simulink model "ROSCO"  (R2023a)
settings: Solver=ode4  StartTime=0.0  StopTime=TMax  FixedStep=simu.dt  RelTol=1e-3  EnableMultiTasking=on
undefined symbols (not defined in the file): A_total, Azimuth_list, B_total, Bd_total, C_total, D_total, Dd_total, DiscIntNeverNeededParam, F, n_FixFrameInputs, n_FixFrameOutputs, n_FixFrameStates2, n_RotTripletInputs, n_RotTripletOutputs, n_RotTripletStates2, new_seq_inp, new_seq_out, new_seq_states, OutList, Parameter, R, rpm2radps, simu, strmatch, uop_total, windspeed_list, wop_total, xop_total, yop_List_total
libraries: simulink x10
(part 5 of 5)

== matlab function ROSCO/MPC/SwitchOP/MATLAB Function ==
  data: windspeed input; A output; A_total parameter; C_total parameter; B_total parameter; D_total parameter; windspeed_list parameter; yop_List_total parameter; xop_total parameter; uop_total parameter; B output; C output; D output; Bd output; Dd output; yop_list output; xop output; uop output; Bd_total parameter; Dd_total parameter; wop_total parameter; wop output
function [A, B, C, D, Bd, Dd, yop_list, xop, uop, wop] = fcn(windspeed, A_total, C_total, B_total, D_total, windspeed_list, yop_List_total, xop_total, uop_total, Bd_total, Dd_total, wop_total)
    index_list = find(windspeed >= windspeed_list);
    if isempty(index_list)
        A = A_total(:, :, 1);
        B = B_total(:, :, 1);
        Bd = Bd_total(:, :, 1);
        C = C_total(:, :, 1);
        D = D_total(:, :, 1);
        Dd = Dd_total(:, :, 1);
        yop_list = yop_List_total(:, :, 1);
        xop = xop_total(:, :, 1);
        uop = uop_total(:, :, 1);
        wop = wop_total(:, :, 1);
    else
        index = index_list(end);
        wspd_num = length(windspeed_list);
        if index == wspd_num
            A = A_total(:, :, wspd_num);
            B = B_total(:, :, wspd_num);
            Bd = Bd_total(:, :, wspd_num);
            C = C_total(:, :, wspd_num);
            D = D_total(:, :, wspd_num);
            Dd = Dd_total(:, :, wspd_num);
            yop_list = yop_List_total(:, :, wspd_num);
            xop = xop_total(:, :, wspd_num);
            uop = uop_total(:, :, wspd_num);
            wop = wop_total(:, :, wspd_num);
        else
            wspd_1 = windspeed - windspeed_list(index);
            wspd_2 = windspeed_list(index+1) - windspeed_list(index);

            A = A_total(:, :, index) + wspd_1 .* (A_total(:, :, index+1) - A_total(:, :, index)) ./ wspd_2;
            B = B_total(:, :, index) + wspd_1 .* (B_total(:, :, index+1) - B_total(:, :, index)) ./ wspd_2;
            Bd = Bd_total(:, :, index) + wspd_1 .* (Bd_total(:, :, index+1) - Bd_total(:, :, index)) ./ wspd_2;
            C = C_total(:, :, index) + wspd_1 .* (C_total(:, :, index+1) - C_total(:, :, index)) ./ wspd_2;
            D = D_total(:, :, index) + wspd_1 .* (D_total(:, :, index+1) - D_total(:, :, index)) ./ wspd_2;
            Dd = Dd_total(:, :, index) + wspd_1 .* (Dd_total(:, :, index+1) - Dd_total(:, :, index)) ./ wspd_2;
            yop_list = yop_List_total(:, :, index) + wspd_1 .* (yop_List_total(:, :, index+1) - yop_List_total(:, :, index)) ./ wspd_2;
            xop = xop_total(:, :, index) + wspd_1 .* (xop_total(:, :, index+1) - xop_total(:, :, index)) ./ wspd_2;
            uop = uop_total(:, :, index) + wspd_1 .* (uop_total(:, :, index+1) - uop_total(:, :, index)) ./ wspd_2;
            wop = wop_total(:, :, index) + wspd_1 .* (wop_total(:, :, index+1) - wop_total(:, :, index)) ./ wspd_2;
        end
    end

end

== matlab function ROSCO/LinearModel_Simulink/SwitchOP/MATLAB Function ==
  data: windspeed input; A output; A_total parameter; C_total parameter; B_total parameter; D_total parameter; windspeed_list parameter; yop_List_total parameter; xop_total parameter; uop_total parameter; B output; C output; D output; Bd output; Dd output; yop_list output; xop output; uop output; Bd_total parameter; Dd_total parameter; wop_total parameter; wop output
function [A, B, C, D, Bd, Dd, yop_list, xop, uop, wop] = fcn(windspeed, A_total, C_total, B_total, D_total, windspeed_list, yop_List_total, xop_total, uop_total, Bd_total, Dd_total, wop_total)
    index_list = find(windspeed >= windspeed_list);
    if isempty(index_list)
        A = A_total(:, :, 1);
        B = B_total(:, :, 1);
        Bd = Bd_total(:, :, 1);
        C = C_total(:, :, 1);
        D = D_total(:, :, 1);
        Dd = Dd_total(:, :, 1);
        yop_list = yop_List_total(:, :, 1);
        xop = xop_total(:, :, 1);
        uop = uop_total(:, :, 1);
        wop = wop_total(:, :, 1);
    else
        index = index_list(end);
        wspd_num = length(windspeed_list);
        if index == wspd_num
            A = A_total(:, :, wspd_num);
            B = B_total(:, :, wspd_num);
            Bd = Bd_total(:, :, wspd_num);
            C = C_total(:, :, wspd_num);
            D = D_total(:, :, wspd_num);
            Dd = Dd_total(:, :, wspd_num);
            yop_list = yop_List_total(:, :, wspd_num);
            xop = xop_total(:, :, wspd_num);
            uop = uop_total(:, :, wspd_num);
            wop = wop_total(:, :, wspd_num);
        else
            wspd_1 = windspeed - windspeed_list(index);
            wspd_2 = windspeed_list(index+1) - windspeed_list(index);

            A = A_total(:, :, index) + wspd_1 .* (A_total(:, :, index+1) - A_total(:, :, index)) ./ wspd_2;
            B = B_total(:, :, index) + wspd_1 .* (B_total(:, :, index+1) - B_total(:, :, index)) ./ wspd_2;
            Bd = Bd_total(:, :, index) + wspd_1 .* (Bd_total(:, :, index+1) - Bd_total(:, :, index)) ./ wspd_2;
            C = C_total(:, :, index) + wspd_1 .* (C_total(:, :, index+1) - C_total(:, :, index)) ./ wspd_2;
            D = D_total(:, :, index) + wspd_1 .* (D_total(:, :, index+1) - D_total(:, :, index)) ./ wspd_2;
            Dd = Dd_total(:, :, index) + wspd_1 .* (Dd_total(:, :, index+1) - Dd_total(:, :, index)) ./ wspd_2;
            yop_list = yop_List_total(:, :, index) + wspd_1 .* (yop_List_total(:, :, index+1) - yop_List_total(:, :, index)) ./ wspd_2;
            xop = xop_total(:, :, index) + wspd_1 .* (xop_total(:, :, index+1) - xop_total(:, :, index)) ./ wspd_2;
            uop = uop_total(:, :, index) + wspd_1 .* (uop_total(:, :, index+1) - uop_total(:, :, index)) ./ wspd_2;
            wop = wop_total(:, :, index) + wspd_1 .* (wop_total(:, :, index+1) - wop_total(:, :, index)) ./ wspd_2;
        end
    end

end

== matlab function ROSCO/MPC/Transverseu/MATLAB Function ==
  data: Azimuth input; n_FixFrameInputs input; n_RotTripletInputs input; delta_u input; new_seq_inp input; delat_u_dq output
function delat_u_dq  = Transverse(Azimuth, n_FixFrameInputs, n_RotTripletInputs, delta_u, new_seq_inp)

% compute azimuth positions of blades:
az = Azimuth*pi/180.0 + 2*pi/3* (0:(3-1)) ; % Eq. 1, azimuth in radians   3个叶片的方位角（弧度），叶片1的方位角为初始方位角

% compute transformation matrices
cos_col = cos(az(:));  % 列向量
sin_col = sin(az(:));

ttv = get_tt_inverse(sin_col, cos_col);     % inverse of tt (computed analytically in function below) 逆矩阵

T1cv = zeros(n_FixFrameInputs+3*n_RotTripletInputs, n_FixFrameInputs+3*n_RotTripletInputs);

T1cv(1:n_FixFrameInputs, 1:n_FixFrameInputs) = eye(n_FixFrameInputs);                % Eq. 21  T1c的逆矩阵

for ii = 1:n_RotTripletInputs
    T1cv(n_FixFrameInputs+1+(ii-1)*3 : n_FixFrameInputs+ii*3, n_FixFrameInputs+1+(ii-1)*3 : n_FixFrameInputs+ii*3) = ttv;
end


% T1o = zeros(n_FixFrameOutputs+3*n_RotTripletOutputs, n_FixFrameOutputs+3*n_RotTripletOutputs);
% 
% T1o(1:n_FixFrameOutputs, 1:n_FixFrameOutputs) = eye(n_FixFrameOutputs);              % Tlo (Eq. 23)  输出相关
% 
% for ii = 1:n_RotTripletOutputs
%     T1o(n_FixFrameOutputs+1+(ii-1)*3 : n_FixFrameOutputs+ii*3, n_FixFrameOutputs+1+(ii-1)*3 : n_FixFrameOutputs+ii*3) = tt;
% end


%% 对u进行转换

delat_u_dq = delta_u .* 0;
delat_u_dq(new_seq_inp, :) = T1cv * delta_u(new_seq_inp);

end



function [ttv] = get_tt_inverse(sin_col, cos_col)

    c1 = cos_col(1);
    c2 = cos_col(2);
    c3 = cos_col(3);
    
    s1 = sin_col(1);
    s2 = sin_col(2);
    s3 = sin_col(3);

    
    ttv = [ c2*s3 - s2*c3,  c3*s1 - s3*c1, c1*s2 - s1*c2
               s2 - s3 ,       s3 - s1,       s1 - s2
               c3 - c2 ,       c1 - c3,       c2 - c1 ] / (1.5*sqrt(3));

    return
end

== matlab function ROSCO/MPC/WindSpeedList ==
  data: windspeed_in input; delta_w_list output; wop input; simu_dt input
function delta_w_list = fcn(windspeed_in, wop, simu_dt)
    Np = 20; 
    Nc = 5;
    DT = 0.001;
    DT_gap = 100;
    delta_w_list = zeros(Np, 1);
    delta_w_list(1) = windspeed_in - wop;  % 假设后续风速不变

end

== matlab function ROSCO/Wind Speed Estimator/Soft Start ==
  settings: updateMethod=DISCRETE  sampleTime=simu.dt
  data: startTime input; out output; endTime input; time input; generic input; actual input
function out = softStart(startTime,endTime,time,generic,actual)

as  = Af_sigma(startTime,endTime);
T   = [time^3,time^2,time,1]';

if time < startTime
    act = 0;
    gen = 1;
elseif time >= startTime && time < endTime
    act = as * T; 
    gen = 1 - as * T;
else
    act = 1;
    gen = 0;
end

out = act*actual + gen*generic;
